simulink library "control_selection"  (R2016b)
settings: Solver=VariableStepAuto  StartTime=0.0  StopTime=10.0  RelTol=1e-3
libraries: momentum_dump_lib x1, pd_control_lib x1
settings Model: Creator=taylorreynolds  LastModifiedBy=evich

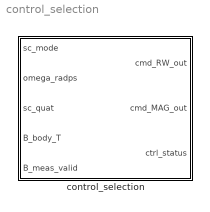
== system control_selection ==
  control_selection : Subsystem

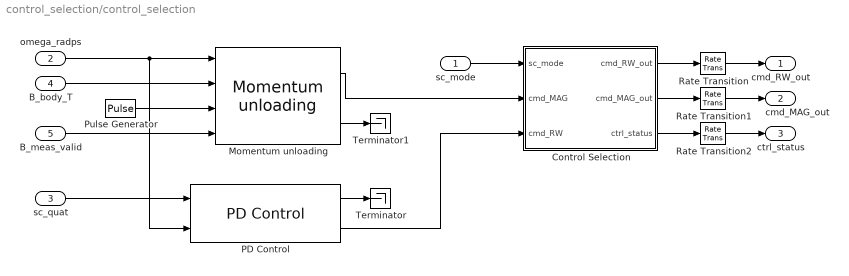
== system control_selection/control_selection ==
  sc_mode : Inport
  omega_radps : Inport  Port=2
  sc_quat : Inport  Port=3
  B_body_T : Inport  Port=4
  B_meas_valid : Inport  Port=5
  Control Selection : Subsystem
  Momentum unloading : momentum_dump_lib/Momentum unloading
  PD Control : pd_control_lib/PD Control
  Pulse Generator : DiscretePulseGenerator  PulseType=Time based  Period=fsw_params.actuators.ppt.sync_pulse  PulseWidth=fsw_params.actuators.ppt.t_charge_pct
  Rate Transition : RateTransition  OutPortSampleTime=fsw_params.sample_time_s
  Rate Transition1 : RateTransition  OutPortSampleTime=fsw_params.sample_time_s
  Rate Transition2 : RateTransition  OutPortSampleTime=fsw_params.sample_time_s
  Terminator : Terminator
  Terminator1 : Terminator
  cmd_RW_out : Outport
  cmd_MAG_out : Outport  Port=2
  ctrl_status : Outport  Port=3
  wires:
  omega_radps/1 -> PD Control/2, Momentum unloading/1
  sc_quat/1 -> PD Control/1
  B_body_T/1 -> Momentum unloading/2
  sc_mode/1 -> Control Selection/1(sc_mode)
  Momentum unloading/1 -> Control Selection/2(cmd_MAG)
  Control Selection/3(ctrl_status) -> Rate Transition2/1
  Control Selection/2("cmd_MAG_out ") -> Rate Transition1/1
  Control Selection/1(cmd_RW_out) -> Rate Transition/1
  PD Control/2 -> Control Selection/3(cmd_RW)
  PD Control/1 -> Terminator/1
  Rate Transition/1 -> cmd_RW_out/1
  Rate Transition2/1 -> ctrl_status/1
  Rate Transition1/1 -> cmd_MAG_out/1
  Pulse Generator/1 -> Momentum unloading/3
  B_meas_valid/1 -> Momentum unloading/4
  Momentum unloading/2 -> Terminator1/1

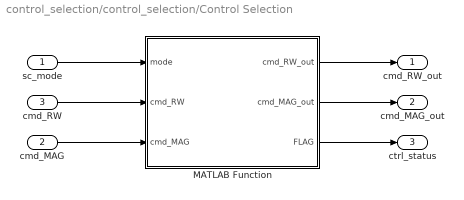
== system control_selection/control_selection/Control Selection ==
  sc_mode : Inport
  cmd_MAG : Inport  Port=2
  cmd_RW : Inport  Port=3
  MATLAB Function : MATLAB Function  TreatAsAtomicUnit=on
  cmd_RW_out : Outport
  "cmd_MAG_out " : Outport  Port=2
  ctrl_status : Outport  Port=3
  wires:
  sc_mode/1 -> MATLAB Function/1(mode)
  cmd_RW/1 -> MATLAB Function/2(cmd_RW)
  cmd_MAG/1 -> MATLAB Function/3(cmd_MAG)
  MATLAB Function/1(cmd_RW_out) -> cmd_RW_out/1
  MATLAB Function/2(cmd_MAG_out) -> "cmd_MAG_out "/1
  MATLAB Function/3(FLAG) -> ctrl_status/1

== matlab function control_selection/Control Selection/MATLAB Function ==
  data: mode input; cmd_RW_out output; cmd_RW input; cmd_MAG input; cmd_MAG_out output; FLAG output
 function [cmd_RW_out,cmd_MAG_out,FLAG] = fcn(mode,cmd_RW,cmd_MAG)
% Control Selection Logic
%   HuskySat-1, ADCS Team
%   Last Update: T. Reynolds, 11.21.17

% Selects which command gets passed to the actuators based on the mode
% provided by upstream mode selection. Current modes are:
%   mode_logic.bdot             = 1;
%   mode_logic.desat_eclipse    = 2;
%   mode_logic.point            = 3;
%       point.velocity          = 31;
%       point.ground            = 32;
%       point.MPC               = 33;
%   mode_logic.low_power        = 4;
%
% FLAG output can be used to make sure the control output matches up with
% what is being commanded, before commands are passed to actuators. FLAG
% should match mode, unless something is wrong.

if mode == 1 
    cmd_RW_out      = zeros(3,1);
    cmd_MAG_out     = zeros(3,1);
    FLAG            = 1;
elseif mode == 2
    cmd_RW_out      = cmd_RW;
    cmd_MAG_out     = cmd_MAG;
    FLAG            = 2;
elseif( mode == 31 || mode == 32 || mode == 33 )
    cmd_RW_out      = cmd_RW;
    cmd_MAG_out     = zeros(3,1);
    FLAG            = mode;
elseif mode == 4
    cmd_RW_out      = zeros(3,1);
    cmd_MAG_out     = zeros(3,1);
    FLAG            = 4;
else
    FLAG = -1;
    cmd_RW_out      = zeros(3,1);
    cmd_MAG_out     = zeros(3,1);
end
